simulink model "Erweiterung"  (R2015a)
settings: Solver=ode45  StartTime=0.0  StopTime=30  RelTol=1e-3
settings Model: Creator=cds-lue-1  LastModifiedBy=cds-lue-1

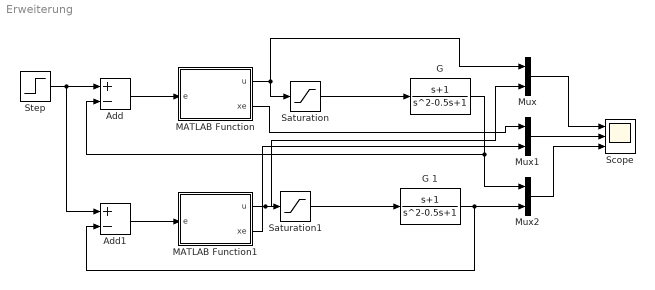
== system Erweiterung ==
  Add : Sum  Inputs=+-
  Add1 : Sum  Inputs=+-
  "G " : TransferFcn  Numerator=[1 1]  Denominator=[1 -0.5 1]
  G 1 : TransferFcn  Numerator=[1 1]  Denominator=[1 -0.5 1]
  MATLAB Function : MATLAB Function  TreatAsAtomicUnit=on  SystemSampleTime=0.001
  MATLAB Function1 : MATLAB Function  TreatAsAtomicUnit=on  SystemSampleTime=0.001
  Mux : Mux  Inputs=2
  Mux1 : Mux  Inputs=2
  Mux2 : Mux  Inputs=2
  Saturation : Saturate  UpperLimit=1  LowerLimit=0
  Saturation1 : Saturate  UpperLimit=1  LowerLimit=0
  Scope : Scope  NumInputPorts=3
      settings: ShowLegends=on  YMin=-5~-5~-5  YMax=5~5~5
  Step : Step  Time=0.1  After=0.9  SampleTime=0
  wires:
  MATLAB Function/1(u) -> Saturation/1, Mux/1
  Saturation/1 -> "G "/1
  Add/1 -> MATLAB Function/1(e)
  Step/1 -> Add1/1, Add/1
  "G "/1 -> Mux2/1, Add/2
  Saturation1/1 -> G 1/1
  MATLAB Function1/1(u) -> Mux/2, Saturation1/1
  Add1/1 -> MATLAB Function1/1(e)
  G 1/1 -> Add1/2, Mux2/2
  Mux2/1 -> Scope/3
  MATLAB Function1/2(xe) -> Mux1/2
  MATLAB Function/2(xe) -> Mux1/1
  Mux1/1 -> Scope/2
  Mux/1 -> Scope/1

== matlab function Erweiterung/MATLAB Function1 ==
  data: u output; e input; xe output
function [u,xe] = fcn(e)
%#codegen
persistent x ;
Ta=0.001;
if(isempty(x))
    x=0;
end

up = 5*e;
ui = 5*x*Ta;

u=up+ui;

if(u<1 && u>0)
    x=x+e;
end
%u=up+ui;
xe=x;

== matlab function Erweiterung/MATLAB Function ==
  data: u output; e input; xe output
function [u,xe] = fcn(e)
%#codegen
persistent x ;
Ta=0.001;
if(isempty(x))
    x=0;
end

up = 5*e;
ui = 5*x;

u=up+ui;

if u>1
    x=(1-up)/5;
end
if u<0
    x=(0-up)/5;
end

if(u<1 && u>0)
    x=x+e*Ta;
end
%u=up+ui;
xe=x;
